simulink model "generic_uservehicle_truck"  (Simulink 10.3)
settings: Solver=ode45  StartTime=0.0  StopTime=inf  RelTol=1e-3  EnableMultiTasking=on
(part 3 of 4)

== system generic_uservehicle_truck/TruckMaker/Vehicle/User Vehicle (CM4SL)/CarAndTrailer/CreateBus Vhcl.Wheel.FL2 ==
  Bus Creator3 : BusCreator  Inputs=14
  Demux3 : Demux  Outputs=14
      settings: DisplayOption=none
  Ground5 : Ground
  Vhcl.Wheel.FL2 : Outport  VectorParamsAs1DForOutWhenUnconnected=off
  wires:
  Demux3/14 -> Bus Creator3/14  "Vhcl Wheel FL2 Trq_WhlBearing"
  Demux3/13 -> Bus Creator3/13  "Vhcl Wheel FL2 Trq_T2W"
  Demux3/12 -> Bus Creator3/12  "Vhcl Wheel FL2 SideSlip"
  Demux3/11 -> Bus Creator3/11  "Vhcl Wheel FL2 LongSlip"
  Demux3/10 -> Bus Creator3/10  "Vhcl Wheel FL2 vBelt"
  Demux3/9 -> Bus Creator3/9  "Vhcl Wheel FL2 Fz"
  Demux3/8 -> Bus Creator3/8  "Vhcl Wheel FL2 Fy"
  Demux3/7 -> Bus Creator3/7  "Vhcl Wheel FL2 Fx"
  Demux3/6 -> Bus Creator3/6  "Vhcl Wheel FL2 r_zxy z"
  Demux3/5 -> Bus Creator3/5  "Vhcl Wheel FL2 r_zxy y"
  Demux3/4 -> Bus Creator3/4  "Vhcl Wheel FL2 r_zxy x"
  Demux3/3 -> Bus Creator3/3  "Vhcl Wheel FL2 t z"
  Demux3/2 -> Bus Creator3/2  "Vhcl Wheel FL2 t y"
  Demux3/1 -> Bus Creator3/1  "Vhcl Wheel FL2 t x"
  Bus Creator3/1 -> Vhcl.Wheel.FL2/1
  Ground5/1 -> Demux3/1

== system generic_uservehicle_truck/TruckMaker/Vehicle/User Vehicle (CM4SL)/CarAndTrailer/CreateBus Vhcl.Wheel.FR ==
  Demux3 : Demux  Outputs=14
      settings: DisplayOption=none
  Ground4 : Ground
  Mux : Mux  Inputs=14
  Vhcl.Wheel.FR : Outport  VectorParamsAs1DForOutWhenUnconnected=off
  wires:
  Demux3/1 -> Mux/1  "Vhcl Wheel FR t x"
  Mux/1 -> Vhcl.Wheel.FR/1
  Ground4/1 -> Demux3/1
  Demux3/2 -> Mux/2  "Vhcl Wheel FR t y"
  Demux3/3 -> Mux/3  "Vhcl Wheel FR t z"
  Demux3/4 -> Mux/4  "Vhcl Wheel FR r_zxy x"
  Demux3/5 -> Mux/5  "Vhcl Wheel FR r_zxy y"
  Demux3/6 -> Mux/6  "Vhcl Wheel FR r_zxy z"
  Demux3/7 -> Mux/7  "Vhcl Wheel FR Fx"
  Demux3/8 -> Mux/8  "Vhcl Wheel FR Fy"
  Demux3/9 -> Mux/9  "Vhcl Wheel FR Fz"
  Demux3/10 -> Mux/10  "Vhcl Wheel FR vBelt"
  Demux3/11 -> Mux/11  "Vhcl Wheel FR LongSlip"
  Demux3/12 -> Mux/12  "Vhcl Wheel FR SideSlip"
  Demux3/13 -> Mux/13  "Vhcl Wheel FR Trq_T2W"
  Demux3/14 -> Mux/14  "Vhcl Wheel FR Trq_WhlBearing"

== system generic_uservehicle_truck/TruckMaker/Vehicle/User Vehicle (CM4SL)/CarAndTrailer/CreateBus Vhcl.Wheel.FR2 ==
  Bus Creator3 : BusCreator  Inputs=14
  Demux3 : Demux  Outputs=14
      settings: DisplayOption=none
  Ground6 : Ground
  Vhcl.Wheel.FR2 : Outport  VectorParamsAs1DForOutWhenUnconnected=off
  wires:
  Demux3/14 -> Bus Creator3/14  "Vhcl Wheel FR2 Trq_WhlBearing"
  Demux3/13 -> Bus Creator3/13  "Vhcl Wheel FR2 Trq_T2W"
  Demux3/12 -> Bus Creator3/12  "Vhcl Wheel FR2 SideSlip"
  Demux3/11 -> Bus Creator3/11  "Vhcl Wheel FR2 LongSlip"
  Demux3/10 -> Bus Creator3/10  "Vhcl Wheel FR2 vBelt"
  Demux3/9 -> Bus Creator3/9  "Vhcl Wheel FR2 Fz"
  Demux3/8 -> Bus Creator3/8  "Vhcl Wheel FR2 Fy"
  Demux3/7 -> Bus Creator3/7  "Vhcl Wheel FR2 Fx"
  Demux3/6 -> Bus Creator3/6  "Vhcl Wheel FR2 r_zxy z"
  Demux3/5 -> Bus Creator3/5  "Vhcl Wheel FR2 r_zxy y"
  Demux3/4 -> Bus Creator3/4  "Vhcl Wheel FR2 r_zxy x"
  Demux3/3 -> Bus Creator3/3  "Vhcl Wheel FR2 t z"
  Demux3/2 -> Bus Creator3/2  "Vhcl Wheel FR2 t y"
  Demux3/1 -> Bus Creator3/1  "Vhcl Wheel FR2 t x"
  Bus Creator3/1 -> Vhcl.Wheel.FR2/1
  Ground6/1 -> Demux3/1

== system generic_uservehicle_truck/TruckMaker/Vehicle/User Vehicle (CM4SL)/CarAndTrailer/CreateBus Vhcl.Wheel.RL ==
  Demux3 : Demux  Outputs=14
      settings: DisplayOption=none
  Ground5 : Ground
  Mux : Mux  Inputs=14
  Vhcl.Wheel.RL : Outport  VectorParamsAs1DForOutWhenUnconnected=off
  wires:
  Demux3/1 -> Mux/1  "Vhcl Wheel RL t x"
  Mux/1 -> Vhcl.Wheel.RL/1
  Ground5/1 -> Demux3/1
  Demux3/2 -> Mux/2  "Vhcl Wheel RL t y"
  Demux3/3 -> Mux/3  "Vhcl Wheel RL t z"
  Demux3/4 -> Mux/4  "Vhcl Wheel RL r_zxy x"
  Demux3/5 -> Mux/5  "Vhcl Wheel RL r_zxy y"
  Demux3/6 -> Mux/6  "Vhcl Wheel RL r_zxy z"
  Demux3/7 -> Mux/7  "Vhcl Wheel RL Fx"
  Demux3/8 -> Mux/8  "Vhcl Wheel RL Fy"
  Demux3/9 -> Mux/9  "Vhcl Wheel RL Fz"
  Demux3/10 -> Mux/10  "Vhcl Wheel RL vBelt"
  Demux3/11 -> Mux/11  "Vhcl Wheel RL LongSlip"
  Demux3/12 -> Mux/12  "Vhcl Wheel RL SideSlip"
  Demux3/13 -> Mux/13  "Vhcl Wheel RL Trq_T2W"
  Demux3/14 -> Mux/14  "Vhcl Wheel RL Trq_WhlBearing"

== system generic_uservehicle_truck/TruckMaker/Vehicle/User Vehicle (CM4SL)/CarAndTrailer/CreateBus Vhcl.Wheel.RL2 ==
  Bus Creator3 : BusCreator  Inputs=14
  Demux3 : Demux  Outputs=14
      settings: DisplayOption=none
  Ground3 : Ground
  Vhcl.Wheel.RL2 : Outport  VectorParamsAs1DForOutWhenUnconnected=off
  wires:
  Bus Creator3/1 -> Vhcl.Wheel.RL2/1
  Demux3/14 -> Bus Creator3/14  "Vhcl Wheel RL2 Trq_WhlBearing"
  Demux3/13 -> Bus Creator3/13  "Vhcl Wheel RL2 Trq_T2W"
  Demux3/12 -> Bus Creator3/12  "Vhcl Wheel RL2 SideSlip"
  Demux3/11 -> Bus Creator3/11  "Vhcl Wheel RL2 LongSlip"
  Demux3/10 -> Bus Creator3/10  "Vhcl Wheel RL2 vBelt"
  Demux3/9 -> Bus Creator3/9  "Vhcl Wheel RL2 Fz"
  Demux3/8 -> Bus Creator3/8  "Vhcl Wheel RL2 Fy"
  Demux3/7 -> Bus Creator3/7  "Vhcl Wheel RL2 Fx"
  Demux3/6 -> Bus Creator3/6  "Vhcl Wheel RL2 r_zxy z"
  Demux3/5 -> Bus Creator3/5  "Vhcl Wheel RL2 r_zxy y"
  Demux3/4 -> Bus Creator3/4  "Vhcl Wheel RL2 r_zxy x"
  Demux3/3 -> Bus Creator3/3  "Vhcl Wheel RL2 t z"
  Demux3/2 -> Bus Creator3/2  "Vhcl Wheel RL2 t y"
  Demux3/1 -> Bus Creator3/1  "Vhcl Wheel RL2 t x"
  Ground3/1 -> Demux3/1

== system generic_uservehicle_truck/TruckMaker/Vehicle/User Vehicle (CM4SL)/CarAndTrailer/CreateBus Vhcl.Wheel.RL3 ==
  Bus Creator3 : BusCreator  Inputs=14
  Demux3 : Demux  Outputs=14
      settings: DisplayOption=none
  Ground3 : Ground
  Vhcl.Wheel.RL3 : Outport  VectorParamsAs1DForOutWhenUnconnected=off
  wires:
  Ground3/1 -> Demux3/1
  Demux3/1 -> Bus Creator3/1  "Vhcl Wheel RL3 t x"
  Demux3/2 -> Bus Creator3/2  "Vhcl Wheel RL3 t y"
  Demux3/3 -> Bus Creator3/3  "Vhcl Wheel RL3 t z"
  Demux3/4 -> Bus Creator3/4  "Vhcl Wheel RL3 r_zxy x"
  Demux3/5 -> Bus Creator3/5  "Vhcl Wheel RL3 r_zxy y"
  Demux3/6 -> Bus Creator3/6  "Vhcl Wheel RL3 r_zxy z"
  Demux3/7 -> Bus Creator3/7  "Vhcl Wheel RL3 Fx"
  Demux3/8 -> Bus Creator3/8  "Vhcl Wheel RL3 Fy"
  Demux3/9 -> Bus Creator3/9  "Vhcl Wheel RL3 Fz"
  Demux3/10 -> Bus Creator3/10  "Vhcl Wheel RL3 vBelt"
  Demux3/11 -> Bus Creator3/11  "Vhcl Wheel RL3 LongSlip"
  Demux3/12 -> Bus Creator3/12  "Vhcl Wheel RL3 SideSlip"
  Demux3/13 -> Bus Creator3/13  "Vhcl Wheel RL3 Trq_T2W"
  Demux3/14 -> Bus Creator3/14  "Vhcl Wheel RL3 Trq_WhlBearing"
  Bus Creator3/1 -> Vhcl.Wheel.RL3/1

== system generic_uservehicle_truck/TruckMaker/Vehicle/User Vehicle (CM4SL)/CarAndTrailer/CreateBus Vhcl.Wheel.RL4 ==
  Bus Creator3 : BusCreator  Inputs=14
  Demux3 : Demux  Outputs=14
      settings: DisplayOption=none
  Ground3 : Ground
  Vhcl.Wheel.RL4 : Outport  VectorParamsAs1DForOutWhenUnconnected=off
  wires:
  Bus Creator3/1 -> Vhcl.Wheel.RL4/1
  Demux3/14 -> Bus Creator3/14  "Vhcl Wheel RL4 Trq_WhlBearing"
  Demux3/13 -> Bus Creator3/13  "Vhcl Wheel RL4 Trq_T2W"
  Demux3/12 -> Bus Creator3/12  "Vhcl Wheel RL4 SideSlip"
  Demux3/11 -> Bus Creator3/11  "Vhcl Wheel RL4 LongSlip"
  Demux3/10 -> Bus Creator3/10  "Vhcl Wheel RL4 vBelt"
  Demux3/9 -> Bus Creator3/9  "Vhcl Wheel RL4 Fz"
  Demux3/8 -> Bus Creator3/8  "Vhcl Wheel RL4 Fy"
  Demux3/7 -> Bus Creator3/7  "Vhcl Wheel RL4 Fx"
  Demux3/6 -> Bus Creator3/6  "Vhcl Wheel RL4 r_zxy z"
  Demux3/5 -> Bus Creator3/5  "Vhcl Wheel RL4 r_zxy y"
  Demux3/4 -> Bus Creator3/4  "Vhcl Wheel RL4 r_zxy x"
  Demux3/3 -> Bus Creator3/3  "Vhcl Wheel RL4 t z"
  Demux3/2 -> Bus Creator3/2  "Vhcl Wheel RL4 t y"
  Demux3/1 -> Bus Creator3/1  "Vhcl Wheel RL4 t x"
  Ground3/1 -> Demux3/1

== system generic_uservehicle_truck/TruckMaker/Vehicle/User Vehicle (CM4SL)/CarAndTrailer/CreateBus Vhcl.Wheel.RR ==
  Demux3 : Demux  Outputs=14
      settings: DisplayOption=none
  Ground6 : Ground
  Mux : Mux  Inputs=14
  Vhcl.Wheel.RR : Outport  VectorParamsAs1DForOutWhenUnconnected=off
  wires:
  Demux3/1 -> Mux/1  "Vhcl Wheel RR t x"
  Mux/1 -> Vhcl.Wheel.RR/1
  Ground6/1 -> Demux3/1
  Demux3/2 -> Mux/2  "Vhcl Wheel RR t y"
  Demux3/3 -> Mux/3  "Vhcl Wheel RR t z"
  Demux3/4 -> Mux/4  "Vhcl Wheel RR r_zxy x"
  Demux3/5 -> Mux/5  "Vhcl Wheel RR r_zxy y"
  Demux3/6 -> Mux/6  "Vhcl Wheel RR r_zxy z"
  Demux3/7 -> Mux/7  "Vhcl Wheel RR Fx"
  Demux3/8 -> Mux/8  "Vhcl Wheel RR Fy"
  Demux3/9 -> Mux/9  "Vhcl Wheel RR Fz"
  Demux3/10 -> Mux/10  "Vhcl Wheel RR vBelt"
  Demux3/11 -> Mux/11  "Vhcl Wheel RR LongSlip"
  Demux3/12 -> Mux/12  "Vhcl Wheel RR SideSlip"
  Demux3/13 -> Mux/13  "Vhcl Wheel RR Trq_T2W"
  Demux3/14 -> Mux/14  "Vhcl Wheel RR Trq_WhlBearing"

== system generic_uservehicle_truck/TruckMaker/Vehicle/User Vehicle (CM4SL)/CarAndTrailer/CreateBus Vhcl.Wheel.RR2 ==
  Bus Creator3 : BusCreator  Inputs=14
  Demux3 : Demux  Outputs=14
      settings: DisplayOption=none
  Ground4 : Ground
  Vhcl.Wheel.RR2 : Outport  VectorParamsAs1DForOutWhenUnconnected=off
  wires:
  Demux3/14 -> Bus Creator3/14  "Vhcl Wheel RR2 Trq_WhlBearing"
  Demux3/13 -> Bus Creator3/13  "Vhcl Wheel RR2 Trq_T2W"
  Demux3/12 -> Bus Creator3/12  "Vhcl Wheel RR2 SideSlip"
  Demux3/11 -> Bus Creator3/11  "Vhcl Wheel RR2 LongSlip"
  Demux3/10 -> Bus Creator3/10  "Vhcl Wheel RR2 vBelt"
  Demux3/9 -> Bus Creator3/9  "Vhcl Wheel RR2 Fz"
  Demux3/8 -> Bus Creator3/8  "Vhcl Wheel RR2 Fy"
  Demux3/7 -> Bus Creator3/7  "Vhcl Wheel RR2 Fx"
  Demux3/6 -> Bus Creator3/6  "Vhcl Wheel RR2 r_zxy z"
  Demux3/5 -> Bus Creator3/5  "Vhcl Wheel RR2 r_zxy y"
  Demux3/4 -> Bus Creator3/4  "Vhcl Wheel RR2 r_zxy x"
  Demux3/3 -> Bus Creator3/3  "Vhcl Wheel RR2 t z"
  Demux3/2 -> Bus Creator3/2  "Vhcl Wheel RR2 t y"
  Demux3/1 -> Bus Creator3/1  "Vhcl Wheel RR2 t x"
  Bus Creator3/1 -> Vhcl.Wheel.RR2/1
  Ground4/1 -> Demux3/1

== system generic_uservehicle_truck/TruckMaker/Vehicle/User Vehicle (CM4SL)/CarAndTrailer/CreateBus Vhcl.Wheel.RR3 ==
  Bus Creator3 : BusCreator  Inputs=14
  Demux3 : Demux  Outputs=14
      settings: DisplayOption=none
  Ground4 : Ground
  Vhcl.Wheel.RR3 : Outport  VectorParamsAs1DForOutWhenUnconnected=off
  wires:
  Ground4/1 -> Demux3/1
  Bus Creator3/1 -> Vhcl.Wheel.RR3/1
  Demux3/1 -> Bus Creator3/1  "Vhcl Wheel RR3 t x"
  Demux3/2 -> Bus Creator3/2  "Vhcl Wheel RR3 t y"
  Demux3/3 -> Bus Creator3/3  "Vhcl Wheel RR3 t z"
  Demux3/4 -> Bus Creator3/4  "Vhcl Wheel RR3 r_zxy x"
  Demux3/5 -> Bus Creator3/5  "Vhcl Wheel RR3 r_zxy y"
  Demux3/6 -> Bus Creator3/6  "Vhcl Wheel RR3 r_zxy z"
  Demux3/7 -> Bus Creator3/7  "Vhcl Wheel RR3 Fx"
  Demux3/8 -> Bus Creator3/8  "Vhcl Wheel RR3 Fy"
  Demux3/9 -> Bus Creator3/9  "Vhcl Wheel RR3 Fz"
  Demux3/10 -> Bus Creator3/10  "Vhcl Wheel RR3 vBelt"
  Demux3/11 -> Bus Creator3/11  "Vhcl Wheel RR3 LongSlip"
  Demux3/12 -> Bus Creator3/12  "Vhcl Wheel RR3 SideSlip"
  Demux3/13 -> Bus Creator3/13  "Vhcl Wheel RR3 Trq_T2W"
  Demux3/14 -> Bus Creator3/14  "Vhcl Wheel RR3 Trq_WhlBearing"

== system generic_uservehicle_truck/TruckMaker/Vehicle/User Vehicle (CM4SL)/CarAndTrailer/CreateBus Vhcl.Wheel.RR4 ==
  Bus Creator3 : BusCreator  Inputs=14
  Demux3 : Demux  Outputs=14
      settings: DisplayOption=none
  Ground4 : Ground
  Vhcl.Wheel.RR4 : Outport  VectorParamsAs1DForOutWhenUnconnected=off
  wires:
  Demux3/14 -> Bus Creator3/14  "Vhcl Wheel RR4 Trq_WhlBearing"
  Demux3/13 -> Bus Creator3/13  "Vhcl Wheel RR4 Trq_T2W"
  Demux3/12 -> Bus Creator3/12  "Vhcl Wheel RR4 SideSlip"
  Demux3/11 -> Bus Creator3/11  "Vhcl Wheel RR4 LongSlip"
  Demux3/10 -> Bus Creator3/10  "Vhcl Wheel RR4 vBelt"
  Demux3/9 -> Bus Creator3/9  "Vhcl Wheel RR4 Fz"
  Demux3/8 -> Bus Creator3/8  "Vhcl Wheel RR4 Fy"
  Demux3/7 -> Bus Creator3/7  "Vhcl Wheel RR4 Fx"
  Demux3/6 -> Bus Creator3/6  "Vhcl Wheel RR4 r_zxy z"
  Demux3/5 -> Bus Creator3/5  "Vhcl Wheel RR4 r_zxy y"
  Demux3/4 -> Bus Creator3/4  "Vhcl Wheel RR4 r_zxy x"
  Demux3/3 -> Bus Creator3/3  "Vhcl Wheel RR4 t z"
  Demux3/2 -> Bus Creator3/2  "Vhcl Wheel RR4 t y"
  Demux3/1 -> Bus Creator3/1  "Vhcl Wheel RR4 t x"
  Bus Creator3/1 -> Vhcl.Wheel.RR4/1
  Ground4/1 -> Demux3/1

== system generic_uservehicle_truck/TruckMaker/Vehicle/User Vehicle (ModelMgr)/Brake/CreateBus Vhcl.Wheel.PT ==
  In : Inport
  BusCreator : BusCreator  Inputs=60
  Demux : Demux  Outputs=60
      settings: DisplayOption=none
  Out : Outport  VectorParamsAs1DForOutWhenUnconnected=off
  wires:
  Demux/60 -> BusCreator/60  "Vhcl Trq_DriveSrc_trg d11"
  Demux/59 -> BusCreator/59  "Vhcl Trq_DriveSrc_trg d10"
  Demux/58 -> BusCreator/58  "Vhcl Trq_DriveSrc_trg d9"
  Demux/57 -> BusCreator/57  "Vhcl Trq_DriveSrc_trg d8"
  Demux/56 -> BusCreator/56  "Vhcl Trq_DriveSrc_trg d7"
  Demux/55 -> BusCreator/55  "Vhcl Trq_DriveSrc_trg d6"
  Demux/54 -> BusCreator/54  "Vhcl Trq_DriveSrc_trg d5"
  Demux/53 -> BusCreator/53  "Vhcl Trq_DriveSrc_trg d4"
  Demux/52 -> BusCreator/52  "Vhcl Trq_DriveSrc_trg d3"
  Demux/51 -> BusCreator/51  "Vhcl Trq_DriveSrc_trg d2"
  Demux/50 -> BusCreator/50  "Vhcl Trq_DriveSrc_trg d1"
  Demux/49 -> BusCreator/49  "Vhcl Trq_DriveSrc_trg d0"
  Demux/48 -> BusCreator/48  "Vhcl Wheel RR4 WhlBearing"
  Demux/47 -> BusCreator/47  "Vhcl Wheel RR4 Trq_T2W"
  Demux/46 -> BusCreator/46  "Vhcl Wheel RR4 Trq_BrakeReg_trg"
  Demux/45 -> BusCreator/45  "Vhcl Wheel RR4 Trq_Brake"
  Demux/44 -> BusCreator/44  "Vhcl Wheel RL4 WhlBearing"
  Demux/43 -> BusCreator/43  "Vhcl Wheel RL4 Trq_T2W"
  Demux/42 -> BusCreator/42  "Vhcl Wheel RL4 Trq_BrakeReg_trg"
  Demux/41 -> BusCreator/41  "Vhcl Wheel RL4 Trq_Brake"
  Demux/40 -> BusCreator/40  "Vhcl Wheel RR3 WhlBearing"
  Demux/39 -> BusCreator/39  "Vhcl Wheel RR3 Trq_T2W"
  Demux/38 -> BusCreator/38  "Vhcl Wheel RR3 Trq_BrakeReg_trg"
  Demux/37 -> BusCreator/37  "Vhcl Wheel RR3 Trq_Brake"
  Demux/36 -> BusCreator/36  "Vhcl Wheel RL3 WhlBearing"
  Demux/35 -> BusCreator/35  "Vhcl Wheel RL3 Trq_T2W"
  Demux/34 -> BusCreator/34  "Vhcl Wheel RL3 Trq_BrakeReg_trg"
  Demux/33 -> BusCreator/33  "Vhcl Wheel RL3 Trq_Brake"
  Demux/32 -> BusCreator/32  "Vhcl Wheel FR2 WhlBearing"
  Demux/31 -> BusCreator/31  "Vhcl Wheel FR2 Trq_T2W"
  Demux/30 -> BusCreator/30  "Vhcl Wheel FR2 Trq_BrakeReg_trg"
  Demux/29 -> BusCreator/29  "Vhcl Wheel FR2 Trq_Brake"
  Demux/28 -> BusCreator/28  "Vhcl Wheel FL2 WhlBearing"
  Demux/27 -> BusCreator/27  "Vhcl Wheel FL2 Trq_T2W"
  Demux/26 -> BusCreator/26  "Vhcl Wheel FL2 Trq_BrakeReg_trg"
  Demux/25 -> BusCreator/25  "Vhcl Wheel FL2 Trq_Brake"
  Demux/24 -> BusCreator/24  "Vhcl Wheel RR2 WhlBearing"
  Demux/23 -> BusCreator/23  "Vhcl Wheel RR2 Trq_T2W"
  Demux/22 -> BusCreator/22  "Vhcl Wheel RR2 Trq_BrakeReg_trg"
  Demux/21 -> BusCreator/21  "Vhcl Wheel RR2 Trq_Brake"
  Demux/20 -> BusCreator/20  "Vhcl Wheel RL2 WhlBearing"
  Demux/19 -> BusCreator/19  "Vhcl Wheel RL2 Trq_T2W"
  Demux/18 -> BusCreator/18  "Vhcl Wheel RL2 Trq_BrakeReg_trg"
  Demux/17 -> BusCreator/17  "Vhcl Wheel RL2 Trq_Brake"
  Demux/16 -> BusCreator/16  "Vhcl Wheel RR WhlBearing"
  Demux/15 -> BusCreator/15  "Vhcl Wheel RR Trq_T2W"
  Demux/14 -> BusCreator/14  "Vhcl Wheel RR Trq_BrakeReg_trg"
  Demux/13 -> BusCreator/13  "Vhcl Wheel RR Trq_Brake"
  Demux/12 -> BusCreator/12  "Vhcl Wheel RL WhlBearing"
  Demux/11 -> BusCreator/11  "Vhcl Wheel RL Trq_T2W"
  Demux/10 -> BusCreator/10  "Vhcl Wheel RL Trq_BrakeReg_trg"
  Demux/9 -> BusCreator/9  "Vhcl Wheel RL Trq_Brake"
  Demux/8 -> BusCreator/8  "Vhcl Wheel FR WhlBearing"
  Demux/7 -> BusCreator/7  "Vhcl Wheel FR Trq_T2W"
  Demux/6 -> BusCreator/6  "Vhcl Wheel FR Trq_BrakeReg_trg"
  Demux/5 -> BusCreator/5  "Vhcl Wheel FR Trq_Brake"
  Demux/4 -> BusCreator/4  "Vhcl Wheel FL WhlBearing"
  Demux/3 -> BusCreator/3  "Vhcl Wheel FL Trq_T2W"
  Demux/2 -> BusCreator/2  "Vhcl Wheel FL Trq_BrakeReg_trg"
  Demux/1 -> BusCreator/1  "Vhcl Wheel FL Trq_Brake"
  BusCreator/1 -> Out/1
  In/1 -> Demux/1

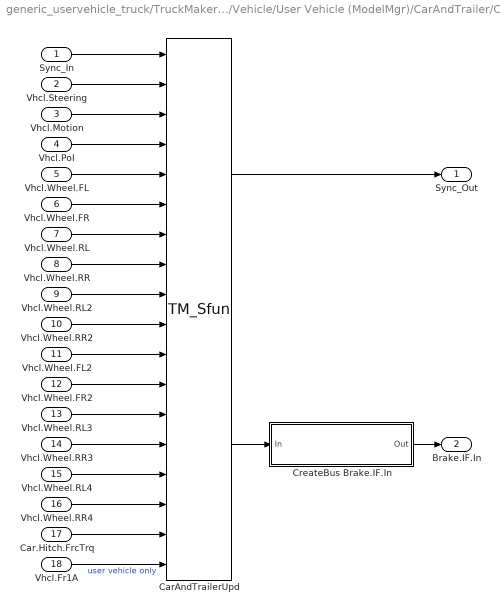
== system generic_uservehicle_truck/TruckMaker/Vehicle/User Vehicle (ModelMgr)/CarAndTrailer/CarAndTrailerUpd ==
  Sync_In : Inport
  Vhcl.Steering : Inport  Port=2
  Vhcl.Motion : Inport  Port=3
  Vhcl.PoI : Inport  Port=4
  Vhcl.Wheel.FL : Inport  Port=5
  Vhcl.Wheel.FR : Inport  Port=6
  Vhcl.Wheel.RL : Inport  Port=7
  Vhcl.Wheel.RR : Inport  Port=8
  Vhcl.Wheel.RL2 : Inport  Port=9
  Vhcl.Wheel.RR2 : Inport  Port=10
  Vhcl.Wheel.FL2 : Inport  Port=11
  Vhcl.Wheel.FR2 : Inport  Port=12
  Vhcl.Wheel.RL3 : Inport  Port=13
  Vhcl.Wheel.RR3 : Inport  Port=14
  Vhcl.Wheel.RL4 : Inport  Port=15
  Vhcl.Wheel.RR4 : Inport  Port=16
  Car.Hitch.FrcTrq : Inport  Port=17
  Vhcl.Fr1A : Inport  Port=18
  CarAndTrailerUpd : S-Function  FunctionName=TM_Sfun  Parameters='CarAndTrUpd'  SFunctionDeploymentMode=off  EnableBusSupport=off
  CreateBus Brake.IF.In : Subsystem
  Sync_Out : Outport  VectorParamsAs1DForOutWhenUnconnected=off
  Brake.IF.In : Outport  Port=2  VectorParamsAs1DForOutWhenUnconnected=off
  wires:
  Vhcl.Wheel.RL3/1 -> CarAndTrailerUpd/13
  Vhcl.Wheel.RR3/1 -> CarAndTrailerUpd/14
  Vhcl.Wheel.RL4/1 -> CarAndTrailerUpd/15
  Vhcl.Wheel.RR4/1 -> CarAndTrailerUpd/16
  Vhcl.Fr1A/1 -> CarAndTrailerUpd/18  "user vehicle only"
  Vhcl.Wheel.RL2/1 -> CarAndTrailerUpd/9
  Vhcl.Wheel.RR2/1 -> CarAndTrailerUpd/10
  Vhcl.Wheel.FL2/1 -> CarAndTrailerUpd/11
  Vhcl.Wheel.FR2/1 -> CarAndTrailerUpd/12
  Car.Hitch.FrcTrq/1 -> CarAndTrailerUpd/17
  Vhcl.Wheel.RR/1 -> CarAndTrailerUpd/8
  Vhcl.Wheel.RL/1 -> CarAndTrailerUpd/7
  Vhcl.Wheel.FR/1 -> CarAndTrailerUpd/6
  Vhcl.Wheel.FL/1 -> CarAndTrailerUpd/5
  Vhcl.Steering/1 -> CarAndTrailerUpd/2
  Vhcl.Motion/1 -> CarAndTrailerUpd/3
  Vhcl.PoI/1 -> CarAndTrailerUpd/4
  CarAndTrailerUpd/2 -> CreateBus Brake.IF.In/1(In)
  CreateBus Brake.IF.In/1(Out) -> Brake.IF.In/1
  CarAndTrailerUpd/1 -> Sync_Out/1
  Sync_In/1 -> CarAndTrailerUpd/1

== system generic_uservehicle_truck/TruckMaker/Vehicle/IPG Vehicle/CarAndTrailer/CarAndTrailerUpd/CreateBus Brake.IF.In ==
  In : Inport
  BusCreator : BusCreator  Inputs=25
  Demux : Demux  Outputs=25
      settings: DisplayOption=none
  Out : Outport  VectorParamsAs1DForOutWhenUnconnected=off
  wires:
  Demux/25 -> BusCreator/25  "Brake IF Trq_Reg RR4"
  Demux/24 -> BusCreator/24  "Brake IF Trq_Reg RL4"
  Demux/23 -> BusCreator/23  "Brake IF Trq_Reg RR3"
  Demux/22 -> BusCreator/22  "Brake IF Trq_Reg RL3"
  Demux/21 -> BusCreator/21  "Brake IF Trq_Reg FR2"
  Demux/20 -> BusCreator/20  "Brake IF Trq_Reg FL2"
  Demux/19 -> BusCreator/19  "Brake IF Trq_Reg RR2"
  Demux/18 -> BusCreator/18  "Brake IF Trq_Reg RL2"
  Demux/17 -> BusCreator/17  "Brake IF Trq_Reg RR"
  Demux/16 -> BusCreator/16  "Brake IF Trq_Reg RL"
  Demux/15 -> BusCreator/15  "Brake IF Trq_Reg FR"
  Demux/14 -> BusCreator/14  "Brake IF Trq_Reg FL"
  Demux/13 -> BusCreator/13  "Brake IF Trq_Reg_max RR4"
  Demux/12 -> BusCreator/12  "Brake IF Trq_Reg_max RL4"
  Demux/11 -> BusCreator/11  "Brake IF Trq_Reg_max RR3"
  Demux/10 -> BusCreator/10  "Brake IF Trq_Reg_max RL3"
  Demux/9 -> BusCreator/9  "Brake IF Trq_Reg_max FR2"
  Demux/8 -> BusCreator/8  "Brake IF Trq_Reg_max FL2"
  Demux/7 -> BusCreator/7  "Brake IF Trq_Reg_max RR2"
  Demux/6 -> BusCreator/6  "Brake IF Trq_Reg_max RL2"
  Demux/5 -> BusCreator/5  "Brake IF Trq_Reg_max RR"
  Demux/4 -> BusCreator/4  "Brake IF Trq_Reg_max RL"
  Demux/3 -> BusCreator/3  "Brake IF Trq_Reg_max FR"
  Demux/2 -> BusCreator/2  "Brake IF Trq_Reg_max FL"
  Demux/1 -> BusCreator/1  "Brake IF T_env"
  BusCreator/1 -> Out/1
  In/1 -> Demux/1

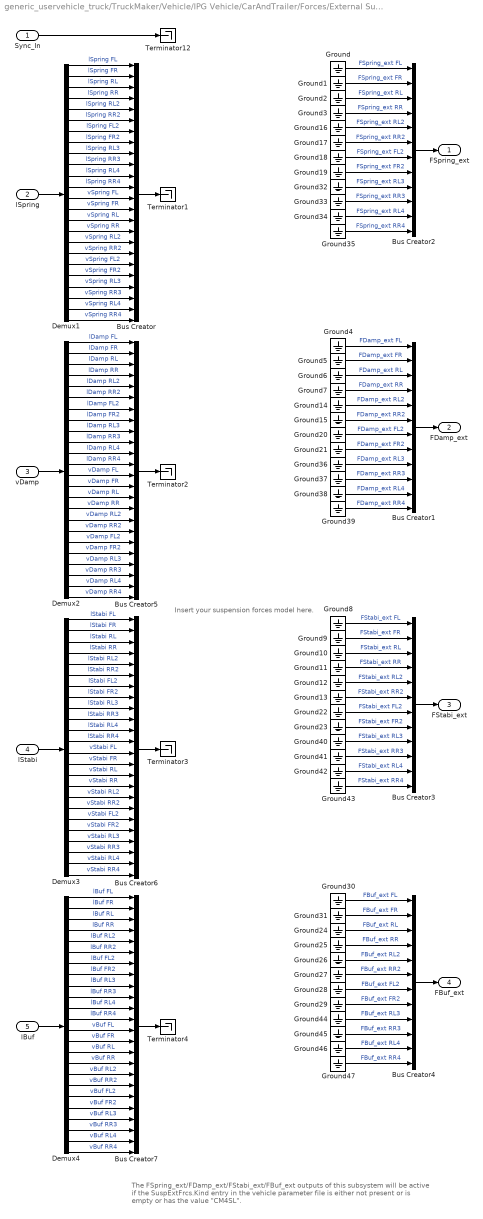
== system generic_uservehicle_truck/TruckMaker/Vehicle/IPG Vehicle/CarAndTrailer/Forces/External Suspension Forces ==
  note: The FSpring_ext/FDamp_ext/FStabi_ext/FBuf_ext outputs of this subsystem will be
      | active if the SuspExtFrcs.Kind entry in the vehicle parameter file
      | is either not present or is empty or has the value "CM4SL".
  note: Insert your suspension forces model here.
  Sync_In : Inport
  lSpring : Inport  Port=2
  vDamp : Inport  Port=3
  lStabi : Inport  Port=4
  lBuf : Inport  Port=5
  Bus Creator{,5..7} (4 alike) : BusCreator  Inputs=24
  Bus Creator{1..4} (4 alike) : BusCreator  Inputs=12
  Demux{1..4} (4 alike) : Demux  Outputs=24
      settings: DisplayOption=none
  Ground{,1..47} (48 alike) : Ground
  Terminator{1..4,12} (5 alike) : Terminator
  FSpring_ext : Outport  VectorParamsAs1DForOutWhenUnconnected=off
  FDamp_ext : Outport  Port=2  VectorParamsAs1DForOutWhenUnconnected=off
  FStabi_ext : Outport  Port=3  VectorParamsAs1DForOutWhenUnconnected=off
  FBuf_ext : Outport  Port=4  VectorParamsAs1DForOutWhenUnconnected=off
  wires:
  Ground46/1 -> Bus Creator4/11  "FBuf_ext RL4"
  Ground47/1 -> Bus Creator4/12  "FBuf_ext RR4"
  Ground45/1 -> Bus Creator4/10  "FBuf_ext RR3"
  Ground44/1 -> Bus Creator4/9  "FBuf_ext RL3"
  Ground42/1 -> Bus Creator3/11  "FStabi_ext RL4"
  Ground43/1 -> Bus Creator3/12  "FStabi_ext RR4"
  Ground41/1 -> Bus Creator3/10  "FStabi_ext RR3"
  Ground40/1 -> Bus Creator3/9  "FStabi_ext RL3"
  Ground38/1 -> Bus Creator1/11  "FDamp_ext RL4"
  Ground39/1 -> Bus Creator1/12  "FDamp_ext RR4"
  Ground37/1 -> Bus Creator1/10  "FDamp_ext RR3"
  Ground36/1 -> Bus Creator1/9  "FDamp_ext RL3"
  Ground35/1 -> Bus Creator2/12  "FSpring_ext RR4"
  Ground34/1 -> Bus Creator2/11  "FSpring_ext RL4"
  Ground33/1 -> Bus Creator2/10  "FSpring_ext RR3"
  Ground32/1 -> Bus Creator2/9  "FSpring_ext RL3"
  Demux4/24 -> Bus Creator7/24  "vBuf RR4"
  Demux4/23 -> Bus Creator7/23  "vBuf RL4"
  Demux4/22 -> Bus Creator7/22  "vBuf RR3"
  Demux4/21 -> Bus Creator7/21  "vBuf RL3"
  Demux4/20 -> Bus Creator7/20  "vBuf FR2"
  Demux4/19 -> Bus Creator7/19  "vBuf FL2"
  Demux4/18 -> Bus Creator7/18  "vBuf RR2"
  Demux4/17 -> Bus Creator7/17  "vBuf RL2"
  Demux3/24 -> Bus Creator6/24  "vStabi RR4"
  Demux3/23 -> Bus Creator6/23  "vStabi RL4"
  Demux3/22 -> Bus Creator6/22  "vStabi RR3"
  Demux3/21 -> Bus Creator6/21  "vStabi RL3"
  Demux3/20 -> Bus Creator6/20  "vStabi FR2"
  Demux3/19 -> Bus Creator6/19  "vStabi FL2"
  Demux3/18 -> Bus Creator6/18  "vStabi RR2"
  Demux3/17 -> Bus Creator6/17  "vStabi RL2"
  Demux2/24 -> Bus Creator5/24  "vDamp RR4"
  Demux2/23 -> Bus Creator5/23  "vDamp RL4"
  Demux2/22 -> Bus Creator5/22  "vDamp RR3"
  Demux2/21 -> Bus Creator5/21  "vDamp RL3"
  Demux2/20 -> Bus Creator5/20  "vDamp FR2"
  Demux2/19 -> Bus Creator5/19  "vDamp FL2"
  Demux2/18 -> Bus Creator5/18  "vDamp RR2"
  Demux2/17 -> Bus Creator5/17  "vDamp RL2"
  Demux1/24 -> Bus Creator/24  "vSpring RR4"
  Demux1/23 -> Bus Creator/23  "vSpring RL4"
  Demux1/22 -> Bus Creator/22  "vSpring RR3"
  Demux1/21 -> Bus Creator/21  "vSpring RL3"
  Demux1/20 -> Bus Creator/20  "vSpring FR2"
  Demux1/19 -> Bus Creator/19  "vSpring FL2"
  Demux1/18 -> Bus Creator/18  "vSpring RR2"
  Demux1/17 -> Bus Creator/17  "vSpring RL2"
  Demux3/10 -> Bus Creator6/10  "lStabi RR3"
  Demux4/16 -> Bus Creator7/16  "vBuf RR"
  Demux4/15 -> Bus Creator7/15  "vBuf RL"
  Demux4/14 -> Bus Creator7/14  "vBuf FR"
  Demux4/13 -> Bus Creator7/13  "vBuf FL"
  Demux4/12 -> Bus Creator7/12  "lBuf RR4"
  Demux4/11 -> Bus Creator7/11  "lBuf RL4"
  Demux4/10 -> Bus Creator7/10  "lBuf RR3"
  Demux4/9 -> Bus Creator7/9  "lBuf RL3"
  Demux3/16 -> Bus Creator6/16  "vStabi RR"
  Demux3/15 -> Bus Creator6/15  "vStabi RL"
  Demux3/14 -> Bus Creator6/14  "vStabi FR"
  Demux3/13 -> Bus Creator6/13  "vStabi FL"
  Demux3/12 -> Bus Creator6/12  "lStabi RR4"
  Demux3/11 -> Bus Creator6/11  "lStabi RL4"
  Demux3/9 -> Bus Creator6/9  "lStabi RL3"
  Bus Creator6/1 -> Terminator3/1
  Bus Creator7/1 -> Terminator4/1
  Bus Creator5/1 -> Terminator2/1
  Bus Creator/1 -> Terminator1/1
  Demux2/16 -> Bus Creator5/16  "vDamp RR"
  Demux2/15 -> Bus Creator5/15  "vDamp RL"
  Demux2/14 -> Bus Creator5/14  "vDamp FR"
  Demux2/13 -> Bus Creator5/13  "vDamp FL"
  Demux2/12 -> Bus Creator5/12  "lDamp RR4"
  Demux2/11 -> Bus Creator5/11  "lDamp RL4"
  Demux2/10 -> Bus Creator5/10  "lDamp RR3"
  Demux2/9 -> Bus Creator5/9  "lDamp RL3"
  Demux1/16 -> Bus Creator/16  "vSpring RR"
  Demux1/15 -> Bus Creator/15  "vSpring RL"
  Demux1/14 -> Bus Creator/14  "vSpring FR"
  Demux1/13 -> Bus Creator/13  "vSpring FL"
  Demux1/12 -> Bus Creator/12  "lSpring RR4"
  Demux1/11 -> Bus Creator/11  "lSpring RL4"
  Demux1/10 -> Bus Creator/10  "lSpring RR3"
  Demux1/9 -> Bus Creator/9  "lSpring RL3"
  Demux3/7 -> Bus Creator6/7  "lStabi FL2"
  Demux3/8 -> Bus Creator6/8  "lStabi FR2"
  Ground22/1 -> Bus Creator3/7  "FStabi_ext FL2"
  Ground23/1 -> Bus Creator3/8  "FStabi_ext FR2"
  Demux2/7 -> Bus Creator5/7  "lDamp FL2"
  Demux2/8 -> Bus Creator5/8  "lDamp FR2"
  Ground20/1 -> Bus Creator1/7  "FDamp_ext FL2"
  Ground21/1 -> Bus Creator1/8  "FDamp_ext FR2"
  Ground18/1 -> Bus Creator2/7  "FSpring_ext FL2"
  Ground19/1 -> Bus Creator2/8  "FSpring_ext FR2"
  Demux1/7 -> Bus Creator/7  "lSpring FL2"
  Demux1/8 -> Bus Creator/8  "lSpring FR2"
  Sync_In/1 -> Terminator12/1
  lSpring/1 -> Demux1/1
  vDamp/1 -> Demux2/1
  lStabi/1 -> Demux3/1
  Demux3/1 -> Bus Creator6/1  "lStabi FL"
  Demux3/2 -> Bus Creator6/2  "lStabi FR"
  Demux3/3 -> Bus Creator6/3  "lStabi RL"
  Demux3/4 -> Bus Creator6/4  "lStabi RR"
  Demux1/1 -> Bus Creator/1  "lSpring FL"
  Demux1/2 -> Bus Creator/2  "lSpring FR"
  Demux1/3 -> Bus Creator/3  "lSpring RL"
  Demux1/4 -> Bus Creator/4  "lSpring RR"
  Demux2/1 -> Bus Creator5/1  "lDamp FL"
  Demux2/2 -> Bus Creator5/2  "lDamp FR"
  Demux2/3 -> Bus Creator5/3  "lDamp RL"
  Demux2/4 -> Bus Creator5/4  "lDamp RR"
  Bus Creator2/1 -> FSpring_ext/1
  Ground/1 -> Bus Creator2/1  "FSpring_ext FL"
  Ground1/1 -> Bus Creator2/2  "FSpring_ext FR"
  Ground2/1 -> Bus Creator2/3  "FSpring_ext RL"
  Ground3/1 -> Bus Creator2/4  "FSpring_ext RR"
  Ground4/1 -> Bus Creator1/1  "FDamp_ext FL"
  Ground5/1 -> Bus Creator1/2  "FDamp_ext FR"
  Ground6/1 -> Bus Creator1/3  "FDamp_ext RL"
  Ground7/1 -> Bus Creator1/4  "FDamp_ext RR"
  Bus Creator1/1 -> FDamp_ext/1
  Ground8/1 -> Bus Creator3/1  "FStabi_ext FL"
  Ground9/1 -> Bus Creator3/2  "FStabi_ext FR"
  Ground10/1 -> Bus Creator3/3  "FStabi_ext RL"
  Ground11/1 -> Bus Creator3/4  "FStabi_ext RR"
  Bus Creator3/1 -> FStabi_ext/1
  Demux3/5 -> Bus Creator6/5  "lStabi RL2"
  Demux3/6 -> Bus Creator6/6  "lStabi RR2"
  Ground12/1 -> Bus Creator3/5  "FStabi_ext RL2"
  Ground13/1 -> Bus Creator3/6  "FStabi_ext RR2"
  Demux2/5 -> Bus Creator5/5  "lDamp RL2"
  Demux2/6 -> Bus Creator5/6  "lDamp RR2"
  Ground14/1 -> Bus Creator1/5  "FDamp_ext RL2"
  Ground15/1 -> Bus Creator1/6  "FDamp_ext RR2"
  Demux1/5 -> Bus Creator/5  "lSpring RL2"
  Demux1/6 -> Bus Creator/6  "lSpring RR2"
  Ground16/1 -> Bus Creator2/5  "FSpring_ext RL2"
  Ground17/1 -> Bus Creator2/6  "FSpring_ext RR2"
  Demux4/7 -> Bus Creator7/7  "lBuf FL2"
  Demux4/8 -> Bus Creator7/8  "lBuf FR2"
  Ground28/1 -> Bus Creator4/7  "FBuf_ext FL2"
  Ground29/1 -> Bus Creator4/8  "FBuf_ext FR2"
  lBuf/1 -> Demux4/1
  Demux4/1 -> Bus Creator7/1  "lBuf FL"
  Demux4/2 -> Bus Creator7/2  "lBuf FR"
  Demux4/3 -> Bus Creator7/3  "lBuf RL"
  Demux4/4 -> Bus Creator7/4  "lBuf RR"
  Ground30/1 -> Bus Creator4/1  "FBuf_ext FL"
  Ground31/1 -> Bus Creator4/2  "FBuf_ext FR"
  Ground24/1 -> Bus Creator4/3  "FBuf_ext RL"
  Ground25/1 -> Bus Creator4/4  "FBuf_ext RR"
  Bus Creator4/1 -> FBuf_ext/1
  Demux4/5 -> Bus Creator7/5  "lBuf RL2"
  Demux4/6 -> Bus Creator7/6  "lBuf RR2"
  Ground26/1 -> Bus Creator4/5  "FBuf_ext RL2"
  Ground27/1 -> Bus Creator4/6  "FBuf_ext RR2"

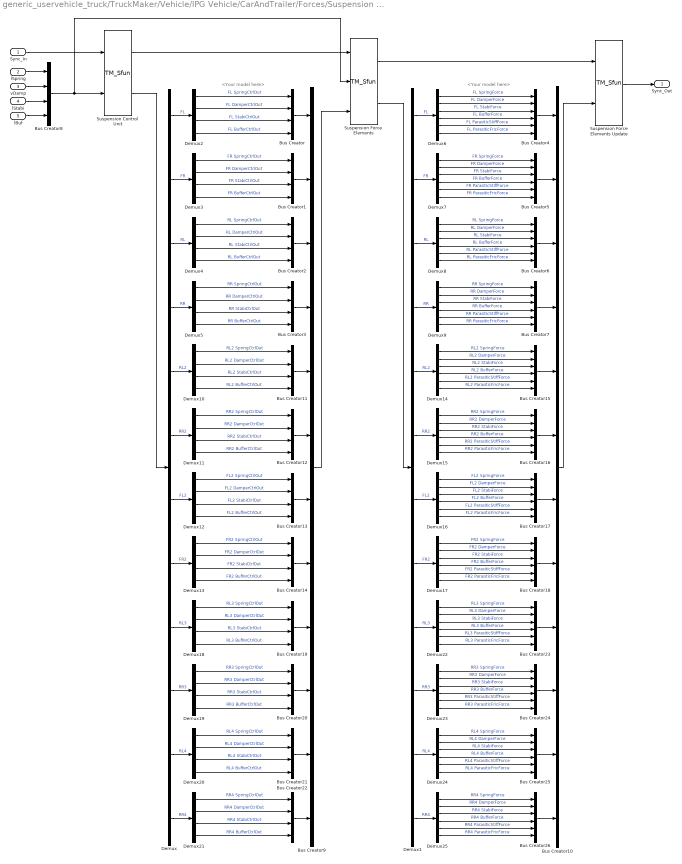
== system generic_uservehicle_truck/TruckMaker/Vehicle/IPG Vehicle/CarAndTrailer/Forces/Suspension Forces ==
  note: <Your model here>
  note: <Your model here>
  Sync_In : Inport
  lSpring : Inport  Port=2
  vDamp : Inport  Port=3
  lStabi : Inport  Port=4
  lBuf : Inport  Port=5
  Bus Creator{,1..3,8,11..14,19..22} (13 alike) : BusCreator  Inputs=4
  Bus Creator10 : BusCreator  Inputs=12
  Bus Creator{4..7,15..18,23..26} (12 alike) : BusCreator  Inputs=6
  Bus Creator9 : BusCreator  Inputs=12
  Demux : Demux  Outputs=12
  Demux1 : Demux  Outputs=12
  Demux{2..5,10..13,18..21} (12 alike) : Demux
  Demux{6..9,14..17,22..25} (12 alike) : Demux  Outputs=6
  Suspension Control Unit : S-Function  FunctionName=TM_Sfun  Parameters='ForcesSuspControl'  SFunctionDeploymentMode=off  EnableBusSupport=off
  Suspension Force Elements : S-Function  FunctionName=TM_Sfun  Parameters='ForcesSusp'  SFunctionDeploymentMode=off  EnableBusSupport=off
  Suspension Force Elements Update : S-Function  FunctionName=TM_Sfun  Parameters='ForcesSuspUpd'  SFunctionDeploymentMode=off  EnableBusSupport=off
  Sync_Out : Outport  VectorParamsAs1DForOutWhenUnconnected=off
  wires:
  Bus Creator26/1 -> Bus Creator10/12
  Bus Creator25/1 -> Bus Creator10/11
  Bus Creator24/1 -> Bus Creator10/10
  Bus Creator23/1 -> Bus Creator10/9
  Demux1/12 -> Demux25/1  "RR4"
  Demux1/11 -> Demux24/1  "RL4"
  Demux1/10 -> Demux23/1  "RR3"
  Demux1/9 -> Demux22/1  "RL3"
  Demux24/6 -> Bus Creator25/6  "RL4 ParasiticFricForce"
  Demux24/5 -> Bus Creator25/5  "RL4 ParasiticStiffForce"
  Demux24/4 -> Bus Creator25/4  "RL4 BufferForce"
  Demux24/3 -> Bus Creator25/3  "RL4 StabiForce"
  Demux24/2 -> Bus Creator25/2  "RL4 DamperForce"
  Demux25/6 -> Bus Creator26/6  "RR4 ParasiticFricForce"
  Demux25/5 -> Bus Creator26/5  "RR4 ParasiticStiffForce"
  Demux25/4 -> Bus Creator26/4  "RR4 BufferForce"
  Demux25/3 -> Bus Creator26/3  "RR4 StabiForce"
  Demux25/2 -> Bus Creator26/2  "RR4 DamperForce"
  Demux25/1 -> Bus Creator26/1  "RR4 SpringForce"
  Demux24/1 -> Bus Creator25/1  "RL4 SpringForce"
  Demux22/1 -> Bus Creator23/1  "RL3 SpringForce"
  Demux23/1 -> Bus Creator24/1  "RR3 SpringForce"
  Demux23/2 -> Bus Creator24/2  "RR3 DamperForce"
  Demux23/3 -> Bus Creator24/3  "RR3 StabiForce"
  Demux23/4 -> Bus Creator24/4  "RR3 BufferForce"
  Demux23/5 -> Bus Creator24/5  "RR3 ParasiticStiffForce"
  Demux23/6 -> Bus Creator24/6  "RR3 ParasiticFricForce"
  Demux22/2 -> Bus Creator23/2  "RL3 DamperForce"
  Demux22/3 -> Bus Creator23/3  "RL3 StabiForce"
  Demux22/4 -> Bus Creator23/4  "RL3 BufferForce"
  Demux22/5 -> Bus Creator23/5  "RL3 ParasiticStiffForce"
  Demux22/6 -> Bus Creator23/6  "RL3 ParasiticFricForce"
  Demux/12 -> Demux21/1  "RR4"
  Demux/11 -> Demux20/1  "RL4"
  Bus Creator21/1 -> Bus Creator9/11
  Demux20/4 -> Bus Creator21/4  "RL4 BufferCtrlOut"
  Demux20/3 -> Bus Creator21/3  "RL4 StabiCtrlOut"
  Demux20/2 -> Bus Creator21/2  "RL4 DamperCtrlOut"
  Demux21/4 -> Bus Creator22/4  "RR4 BufferCtrlOut"
  Demux21/3 -> Bus Creator22/3  "RR4 StabiCtrlOut"
  Demux21/2 -> Bus Creator22/2  "RR4 DamperCtrlOut"
  Demux21/1 -> Bus Creator22/1  "RR4 SpringCtrlOut"
  Demux20/1 -> Bus Creator21/1  "RL4 SpringCtrlOut"
  Bus Creator22/1 -> Bus Creator9/12
  Demux/9 -> Demux18/1  "RL3"
  Bus Creator20/1 -> Bus Creator9/10
  Demux/10 -> Demux19/1  "RR3"
  Demux18/1 -> Bus Creator19/1  "RL3 SpringCtrlOut"
  Demux19/1 -> Bus Creator20/1  "RR3 SpringCtrlOut"
  Demux19/2 -> Bus Creator20/2  "RR3 DamperCtrlOut"
  Demux19/3 -> Bus Creator20/3  "RR3 StabiCtrlOut"
  Demux19/4 -> Bus Creator20/4  "RR3 BufferCtrlOut"
  Demux18/2 -> Bus Creator19/2  "RL3 DamperCtrlOut"
  Demux18/3 -> Bus Creator19/3  "RL3 StabiCtrlOut"
  Demux18/4 -> Bus Creator19/4  "RL3 BufferCtrlOut"
  Bus Creator19/1 -> Bus Creator9/9
  Demux1/8 -> Demux17/1  "FR2"
  Demux1/7 -> Demux16/1  "FL2"
  Demux1/6 -> Demux15/1  "RR2"
  Demux1/5 -> Demux14/1  "RL2"
  Demux14/6 -> Bus Creator15/6  "RL2 ParasiticFricForce"
  Demux14/5 -> Bus Creator15/5  "RL2 ParasiticStiffForce"
  Demux14/4 -> Bus Creator15/4  "RL2 BufferForce"
  Demux14/3 -> Bus Creator15/3  "RL2 StabiForce"
  Demux14/2 -> Bus Creator15/2  "RL2 DamperForce"
  Demux15/6 -> Bus Creator16/6  "RR2 ParasiticFricForce"
  Demux15/5 -> Bus Creator16/5  "RR2 ParasiticStiffForce"
  Demux15/4 -> Bus Creator16/4  "RR2 BufferForce"
  Demux15/3 -> Bus Creator16/3  "RR2 StabiForce"
  Demux15/2 -> Bus Creator16/2  "RR2 DamperForce"
  Demux15/1 -> Bus Creator16/1  "RR2 SpringForce"
  Demux16/3 -> Bus Creator17/3  "FL2 StabiForce"
  Demux16/6 -> Bus Creator17/6  "FL2 ParasiticFricForce"
  Demux16/5 -> Bus Creator17/5  "FL2 ParasiticStiffForce"
  Demux16/4 -> Bus Creator17/4  "FL2 BufferForce"
  Demux16/2 -> Bus Creator17/2  "FL2 DamperForce"
  Demux16/1 -> Bus Creator17/1  "FL2 SpringForce"
  Demux17/6 -> Bus Creator18/6  "FR2 ParasiticFricForce"
  Demux17/5 -> Bus Creator18/5  "FR2 ParasiticStiffForce"
  Demux17/4 -> Bus Creator18/4  "FR2 BufferForce"
  Demux17/3 -> Bus Creator18/3  "FR2 StabiForce"
  Demux17/2 -> Bus Creator18/2  "FR2 DamperForce"
  Demux17/1 -> Bus Creator18/1  "FR2 SpringForce"
  Demux14/1 -> Bus Creator15/1  "RL2 SpringForce"
  Bus Creator18/1 -> Bus Creator10/8
  Bus Creator17/1 -> Bus Creator10/7
  Bus Creator16/1 -> Bus Creator10/6
  Bus Creator15/1 -> Bus Creator10/5
  Bus Creator11/1 -> Bus Creator9/5
  Demux10/4 -> Bus Creator11/4  "RL2 BufferCtrlOut"
  Demux10/3 -> Bus Creator11/3  "RL2 StabiCtrlOut"
  Demux10/2 -> Bus Creator11/2  "RL2 DamperCtrlOut"
  Demux11/4 -> Bus Creator12/4  "RR2 BufferCtrlOut"
  Demux11/3 -> Bus Creator12/3  "RR2 StabiCtrlOut"
  Demux11/2 -> Bus Creator12/2  "RR2 DamperCtrlOut"
  Demux11/1 -> Bus Creator12/1  "RR2 SpringCtrlOut"
  Demux12/3 -> Bus Creator13/3  "FL2 StabiCtrlOut"
  Demux12/4 -> Bus Creator13/4  "FL2 BufferCtrlOut"
  Demux12/2 -> Bus Creator13/2  "FL2 DamperCtrlOut"
  Demux12/1 -> Bus Creator13/1  "FL2 SpringCtrlOut"
  Demux13/4 -> Bus Creator14/4  "FR2 BufferCtrlOut"
  Demux13/3 -> Bus Creator14/3  "FR2 StabiCtrlOut"
  Demux13/2 -> Bus Creator14/2  "FR2 DamperCtrlOut"
  Demux13/1 -> Bus Creator14/1  "FR2 SpringCtrlOut"
  Demux/8 -> Demux13/1  "FR2"
  Demux10/1 -> Bus Creator11/1  "RL2 SpringCtrlOut"
  Bus Creator14/1 -> Bus Creator9/8
  Demux/7 -> Demux12/1  "FL2"
  Bus Creator13/1 -> Bus Creator9/7
  Demux/6 -> Demux11/1  "RR2"
  Bus Creator12/1 -> Bus Creator9/6
  Demux/5 -> Demux10/1  "RL2"
  Demux1/4 -> Demux9/1  "RR"
  Demux1/3 -> Demux8/1  "RL"
  Demux1/2 -> Demux7/1  "FR"
  Demux1/1 -> Demux6/1  "FL"
  Suspension Force Elements/2 -> Demux1/1
  Bus Creator/1 -> Bus Creator9/1
  Bus Creator9/1 -> Suspension Force Elements/3
  Suspension Control Unit/2 -> Demux/1
  Demux2/4 -> Bus Creator/4  "FL BufferCtrlOut"
  Demux2/3 -> Bus Creator/3  "FL StabiCtrlOut"
  Demux2/2 -> Bus Creator/2  "FL DamperCtrlOut"
  Demux3/4 -> Bus Creator1/4  "FR BufferCtrlOut"
  Demux3/3 -> Bus Creator1/3  "FR StabiCtrlOut"
  Demux3/2 -> Bus Creator1/2  "FR DamperCtrlOut"
  Demux3/1 -> Bus Creator1/1  "FR SpringCtrlOut"
  Demux4/3 -> Bus Creator2/3  "RL StabiCtrlOut"
  Demux4/4 -> Bus Creator2/4  "RL BufferCtrlOut"
  Demux4/2 -> Bus Creator2/2  "RL DamperCtrlOut"
  Demux4/1 -> Bus Creator2/1  "RL SpringCtrlOut"
  Demux5/4 -> Bus Creator3/4  "RR BufferCtrlOut"
  Demux5/3 -> Bus Creator3/3  "RR StabiCtrlOut"
  Demux5/2 -> Bus Creator3/2  "RR DamperCtrlOut"
  Demux5/1 -> Bus Creator3/1  "RR SpringCtrlOut"
  Demux/4 -> Demux5/1  "RR"
  Demux2/1 -> Bus Creator/1  "FL SpringCtrlOut"
  Bus Creator3/1 -> Bus Creator9/4
  Demux/3 -> Demux4/1  "RL"
  Bus Creator2/1 -> Bus Creator9/3
  Demux/2 -> Demux3/1  "FR"
  Bus Creator1/1 -> Bus Creator9/2
  Demux/1 -> Demux2/1  "FL"
  Bus Creator10/1 -> Suspension Force Elements Update/2
  Demux6/6 -> Bus Creator4/6  "FL ParasiticFricForce"
  Demux6/5 -> Bus Creator4/5  "FL ParasiticStiffForce"
  Demux6/4 -> Bus Creator4/4  "FL BufferForce"
  Demux6/3 -> Bus Creator4/3  "FL StabiForce"
  Demux6/2 -> Bus Creator4/2  "FL DamperForce"
  Demux7/6 -> Bus Creator5/6  "FR ParasiticFricForce"
  Demux7/5 -> Bus Creator5/5  "FR ParasiticStiffForce"
  Demux7/4 -> Bus Creator5/4  "FR BufferForce"
  Demux7/3 -> Bus Creator5/3  "FR StabiForce"
  Demux7/2 -> Bus Creator5/2  "FR DamperForce"
  Demux7/1 -> Bus Creator5/1  "FR SpringForce"
  Demux8/3 -> Bus Creator6/3  "RL StabiForce"
  Demux8/6 -> Bus Creator6/6  "RL ParasiticFricForce"
  Demux8/5 -> Bus Creator6/5  "RL ParasiticStiffForce"
  Demux8/4 -> Bus Creator6/4  "RL BufferForce"
  Demux8/2 -> Bus Creator6/2  "RL DamperForce"
  Demux8/1 -> Bus Creator6/1  "RL SpringForce"
  Demux9/6 -> Bus Creator7/6  "RR ParasiticFricForce"
  Demux9/5 -> Bus Creator7/5  "RR ParasiticStiffForce"
  Demux9/4 -> Bus Creator7/4  "RR BufferForce"
  Demux9/3 -> Bus Creator7/3  "RR StabiForce"
  Demux9/2 -> Bus Creator7/2  "RR DamperForce"
  Demux9/1 -> Bus Creator7/1  "RR SpringForce"
  Demux6/1 -> Bus Creator4/1  "FL SpringForce"
  Bus Creator7/1 -> Bus Creator10/4
  Bus Creator6/1 -> Bus Creator10/3
  Bus Creator5/1 -> Bus Creator10/2
  Bus Creator4/1 -> Bus Creator10/1
  Suspension Force Elements Update/1 -> Sync_Out/1
  Suspension Force Elements/1 -> Suspension Force Elements Update/1
  Suspension Control Unit/1 -> Suspension Force Elements/1
  Sync_In/1 -> Suspension Control Unit/1
  Bus Creator8/1 -> Suspension Force Elements/2, Suspension Control Unit/2
  lSpring/1 -> Bus Creator8/1
  lBuf/1 -> Bus Creator8/4
  lStabi/1 -> Bus Creator8/3
  vDamp/1 -> Bus Creator8/2

== system generic_uservehicle_truck/TruckMaker/Vehicle/IPG Vehicle/CarAndTrailer/Forces/Vehicle Forces ==
  Sync_In : Inport
  Bus Creator1 : BusCreator  Inputs=12
  Bus Creator8 : BusCreator  Inputs=16
  BusCreator1 : BusCreator  Inputs=4
  BusCreator2 : BusCreator  Inputs=9
  Demux : Demux  Outputs=16
      settings: DisplayOption=none
  Demux1 : Demux  Outputs=12
      settings: DisplayOption=none
  Demux2 : Demux  Outputs=13
      settings: DisplayOption=none
  Forces : S-Function  FunctionName=TM_Sfun  Parameters='Forces'  SFunctionDeploymentMode=off  EnableBusSupport=off
  Terminator : Terminator
  Sync_Out : Outport  VectorParamsAs1DForOutWhenUnconnected=off
  Car.Virtual : Outport  Port=2  VectorParamsAs1DForOutWhenUnconnected=off
  Car.Aero : Outport  Port=3  VectorParamsAs1DForOutWhenUnconnected=off
  Car.Load : Outport  Port=4  VectorParamsAs1DForOutWhenUnconnected=off
  wires:
  BusCreator1/1 -> Terminator/1  "Aero IF (in)"
  Demux2/13 -> BusCreator2/9  "car Aero Trq_1 z"
  Demux2/12 -> BusCreator2/8  "car Aero Trq_1 y"
  Demux2/11 -> BusCreator2/7  "car Aero Trq_1 x"
  Demux2/10 -> BusCreator2/6  "car Aero Frc_1 z"
  Demux2/9 -> BusCreator2/5  "car Aero Frc_1 y"
  Demux2/8 -> BusCreator2/4  "car Aero Frc_1 x"
  Demux2/7 -> BusCreator2/3  "car Aero PoA_1 z"
  Demux2/6 -> BusCreator2/2  "car Aero PoA_1 y"
  Demux2/5 -> BusCreator2/1  "car Aero PoA_1 x"
  Demux2/4 -> BusCreator1/4  "car Aero tau_1"
  Demux2/3 -> BusCreator1/3  "car Aero ApproachVel_1 z"
  Demux2/2 -> BusCreator1/2  "car Aero ApproachVel_1 y"
  Demux2/1 -> BusCreator1/1  "car Aero ApproachVel_1 x"
  BusCreator2/1 -> Car.Aero/1
  Demux/16 -> Bus Creator8/16  "Car Load_3 tz"
  Demux/15 -> Bus Creator8/15  "Car Load_3 ty"
  Demux/14 -> Bus Creator8/14  "Car Load_3 tx"
  Demux/13 -> Bus Creator8/13  "Car Load_3 mass"
  Demux1/12 -> Bus Creator1/12  "Car Virtual Trq_0 z"
  Demux1/11 -> Bus Creator1/11  "Car Virtual Trq_0 y"
  Demux1/10 -> Bus Creator1/10  "Car Virtual Trq_0 x"
  Demux1/9 -> Bus Creator1/9  "Car Virtual Trq_1 z"
  Demux1/8 -> Bus Creator1/8  "Car Virtual Trq_1 y"
  Demux1/7 -> Bus Creator1/7  "Car Virtual Trq_1 x"
  Demux1/6 -> Bus Creator1/6  "Car Virtual Frc_0 z"
  Demux1/5 -> Bus Creator1/5  "Car Virtual Frc_0 y"
  Demux1/4 -> Bus Creator1/4  "Car Virtual Frc_0 x"
  Sync_In/1 -> Forces/1
  Forces/1 -> Sync_Out/1
  Demux1/1 -> Bus Creator1/1  "Car Virtual Frc_1 x"
  Demux1/2 -> Bus Creator1/2  "Car Virtual Frc_1 y"
  Demux1/3 -> Bus Creator1/3  "Car Virtual Frc_1 z"
  Forces/3 -> Demux2/1
  Forces/2 -> Demux1/1
  Bus Creator1/1 -> Car.Virtual/1
  Bus Creator8/1 -> Car.Load/1
  Demux/1 -> Bus Creator8/1  "Car Load_0 mass"
  Demux/2 -> Bus Creator8/2  "Car Load_0 tx"
  Demux/3 -> Bus Creator8/3  "Car Load_0 ty"
  Demux/4 -> Bus Creator8/4  "Car Load_0 tz"
  Demux/5 -> Bus Creator8/5  "Car Load_1 mass"
  Demux/6 -> Bus Creator8/6  "Car Load_1 tx"
  Demux/7 -> Bus Creator8/7  "Car Load_1 ty"
  Demux/8 -> Bus Creator8/8  "Car Load_1 tz"
  Demux/9 -> Bus Creator8/9  "Car Load_2 mass"
  Demux/10 -> Bus Creator8/10  "Car Load_2 tx"
  Demux/11 -> Bus Creator8/11  "Car Load_2 ty"
  Demux/12 -> Bus Creator8/12  "Car Load_2 tz"
  Forces/4 -> Demux/1

== system generic_uservehicle_truck/TruckMaker/Vehicle/IPG Vehicle/CarAndTrailer/Trailer/CreateBus Car.Hitch.FrcTrq ==
  In1 : Inport
  Bus Creator7 : BusCreator  Inputs=6
  Demux7 : Demux  Outputs=6
      settings: DisplayOption=none
  Out1 : Outport  VectorParamsAs1DForOutWhenUnconnected=off
  wires:
  In1/1 -> Demux7/1
  Bus Creator7/1 -> Out1/1
  Demux7/6 -> Bus Creator7/6  "Car Hitch Trq2Car z"
  Demux7/5 -> Bus Creator7/5  "Car Hitch Trq2Car y"
  Demux7/4 -> Bus Creator7/4  "Car Hitch Trq2Car x"
  Demux7/3 -> Bus Creator7/3  "Car Hitch Frc2Car z"
  Demux7/2 -> Bus Creator7/2  "Car Hitch Frc2Car y"
  Demux7/1 -> Bus Creator7/1  "Car Hitch Frc2Car x"

== system generic_uservehicle_truck/TruckMaker/Vehicle/IPG Vehicle/CarAndTrailer/Trailer/CreateBus Vhcl.Motion ==
  In1 : Inport
  BusCreator : BusCreator  Inputs=15
  Demux : Demux  Outputs=15
      settings: DisplayOption=none
  Out1 : Outport  VectorParamsAs1DForOutWhenUnconnected=off
  wires:
  Demux/15 -> BusCreator/15  "Vhcl YawAcc"
  Demux/14 -> BusCreator/14  "Vhcl YawVel"
  Demux/13 -> BusCreator/13  "Vhcl Yaw"
  Demux/12 -> BusCreator/12  "Vhcl PitchAcc"
  Demux/11 -> BusCreator/11  "Vhcl PitchVel"
  Demux/10 -> BusCreator/10  "Vhcl Pitch"
  Demux/9 -> BusCreator/9  "Vhcl RollAcc"
  Demux/8 -> BusCreator/8  "Vhcl RollVel"
  Demux/7 -> BusCreator/7  "Vhcl Roll"
  Demux/6 -> BusCreator/6  "Vhcl Hitch_Pos z"
  Demux/5 -> BusCreator/5  "Vhcl Hitch_Pos y"
  Demux/4 -> BusCreator/4  "Vhcl Hitch_Pos x"
  Demux/3 -> BusCreator/3  "Vhcl sRoad"
  Demux/2 -> BusCreator/2  "Vhcl Distance"
  Demux/1 -> BusCreator/1  "Vhcl v"
  In1/1 -> Demux/1
  BusCreator/1 -> Out1/1

== system generic_uservehicle_truck/TruckMaker/Vehicle/IPG Vehicle/CarAndTrailer/Trailer/CreateBus Vhcl.PoI ==
  In1 : Inport
  Bus Creator3 : BusCreator  Inputs=18
  Demux3 : Demux  Outputs=18
      settings: DisplayOption=none
  Out1 : Outport  VectorParamsAs1DForOutWhenUnconnected=off
  wires:
  Demux3/18 -> Bus Creator3/18  "Vhcl PoI_GCS Elev"
  Demux3/17 -> Bus Creator3/17  "Vhcl PoI_GCS Lat"
  Demux3/16 -> Bus Creator3/16  "Vhcl PoI_GCS Long"
  Demux3/15 -> Bus Creator3/15  "Vhcl PoI_Acc_1 z"
  Demux3/14 -> Bus Creator3/14  "Vhcl PoI_Acc_1 y"
  Demux3/13 -> Bus Creator3/13  "Vhcl PoI_Acc_1 x"
  Demux3/12 -> Bus Creator3/12  "Vhcl PoI_Vel_1 z"
  Demux3/11 -> Bus Creator3/11  "Vhcl PoI_Vel_1 y"
  Demux3/10 -> Bus Creator3/10  "Vhcl PoI_Vel_1 x"
  Demux3/9 -> Bus Creator3/9  "Vhcl PoI_Acc z"
  Demux3/8 -> Bus Creator3/8  "Vhcl PoI_Acc y"
  Demux3/7 -> Bus Creator3/7  "Vhcl PoI_Acc x"
  Demux3/6 -> Bus Creator3/6  "Vhcl PoI_Vel z"
  Demux3/5 -> Bus Creator3/5  "Vhcl PoI_Vel y"
  Demux3/4 -> Bus Creator3/4  "Vhcl PoI_Vel x"
  Demux3/3 -> Bus Creator3/3  "Vhcl PoI_Pos z"
  Demux3/2 -> Bus Creator3/2  "Vhcl PoI_Pos y"
  In1/1 -> Demux3/1
  Bus Creator3/1 -> Out1/1
  Demux3/1 -> Bus Creator3/1  "Vhcl PoI_Pos x"

== system generic_uservehicle_truck/TruckMaker/Vehicle/IPG Vehicle/CarAndTrailer/Trailer/CreateBus Vhcl.Steering ==
  In1 : Inport
  Bus Creator3 : BusCreator  Inputs=4
  Demux : Demux
      settings: DisplayOption=none
  Out1 : Outport  VectorParamsAs1DForOutWhenUnconnected=off
  wires:
  Bus Creator3/1 -> Out1/1
  Demux/1 -> Bus Creator3/1  "Vhcl Steering Ang"
  Demux/3 -> Bus Creator3/3  "Vhcl Steering AngAcc"
  Demux/2 -> Bus Creator3/2  "Vhcl Steering AngVel"
  Demux/4 -> Bus Creator3/4  "Vhcl Steering Trq"
  In1/1 -> Demux/1

== system generic_uservehicle_truck/TruckMaker/Vehicle/IPG Vehicle/CarAndTrailer/Trailer/CreateBus Vhcl.Wheel.FL ==
  In1 : Inport
  Bus Creator3 : BusCreator  Inputs=14
  Demux3 : Demux  Outputs=14
      settings: DisplayOption=none
  Out1 : Outport  VectorParamsAs1DForOutWhenUnconnected=off
  wires:
  Demux3/14 -> Bus Creator3/14  "Vhcl Wheel FL Trq_WhlBearing"
  Demux3/13 -> Bus Creator3/13  "Vhcl Wheel FL Trq_T2W"
  Demux3/12 -> Bus Creator3/12  "Vhcl Wheel FL SideSlip"
  Demux3/11 -> Bus Creator3/11  "Vhcl Wheel FL LongSlip"
  Demux3/10 -> Bus Creator3/10  "Vhcl Wheel FL vBelt"
  Demux3/9 -> Bus Creator3/9  "Vhcl Wheel FL Fz"
  Demux3/8 -> Bus Creator3/8  "Vhcl Wheel FL Fy"
  Demux3/7 -> Bus Creator3/7  "Vhcl Wheel FL Fx"
  Demux3/6 -> Bus Creator3/6  "Vhcl Wheel FL r_zxy z"
  Demux3/5 -> Bus Creator3/5  "Vhcl Wheel FL r_zxy y"
  Demux3/4 -> Bus Creator3/4  "Vhcl Wheel FL r_zxy x"
  Demux3/3 -> Bus Creator3/3  "Vhcl Wheel FL t z"
  Demux3/2 -> Bus Creator3/2  "Vhcl Wheel FL t y"
  In1/1 -> Demux3/1
  Bus Creator3/1 -> Out1/1
  Demux3/1 -> Bus Creator3/1  "Vhcl Wheel FL t x"

== system generic_uservehicle_truck/TruckMaker/Vehicle/IPG Vehicle/CarAndTrailer/Trailer/CreateBus Vhcl.Wheel.FL2 ==
  In1 : Inport
  Bus Creator3 : BusCreator  Inputs=14
  Demux3 : Demux  Outputs=14
      settings: DisplayOption=none
  Out1 : Outport  VectorParamsAs1DForOutWhenUnconnected=off
  wires:
  Demux3/14 -> Bus Creator3/14  "Vhcl Wheel FL2 Trq_WhlBearing"
  Demux3/13 -> Bus Creator3/13  "Vhcl Wheel FL2 Trq_T2W"
  Demux3/12 -> Bus Creator3/12  "Vhcl Wheel FL2 SideSlip"
  Demux3/11 -> Bus Creator3/11  "Vhcl Wheel FL2 LongSlip"
  Demux3/10 -> Bus Creator3/10  "Vhcl Wheel FL2 vBelt"
  Demux3/9 -> Bus Creator3/9  "Vhcl Wheel FL2 Fz"
  Demux3/8 -> Bus Creator3/8  "Vhcl Wheel FL2 Fy"
  Demux3/7 -> Bus Creator3/7  "Vhcl Wheel FL2 Fx"
  Demux3/6 -> Bus Creator3/6  "Vhcl Wheel FL2 r_zxy z"
  Demux3/5 -> Bus Creator3/5  "Vhcl Wheel FL2 r_zxy y"
  Demux3/4 -> Bus Creator3/4  "Vhcl Wheel FL2 r_zxy x"
  Demux3/3 -> Bus Creator3/3  "Vhcl Wheel FL2 t z"
  Demux3/2 -> Bus Creator3/2  "Vhcl Wheel FL2 t y"
  In1/1 -> Demux3/1
  Bus Creator3/1 -> Out1/1
  Demux3/1 -> Bus Creator3/1  "Vhcl Wheel FL2 t x"

== system generic_uservehicle_truck/TruckMaker/Vehicle/IPG Vehicle/CarAndTrailer/Trailer/CreateBus Vhcl.Wheel.FR ==
  In1 : Inport
  Bus Creator3 : BusCreator  Inputs=14
  Demux3 : Demux  Outputs=14
      settings: DisplayOption=none
  Out1 : Outport  VectorParamsAs1DForOutWhenUnconnected=off
  wires:
  Demux3/14 -> Bus Creator3/14  "Vhcl Wheel FR Trq_WhlBearing"
  Demux3/13 -> Bus Creator3/13  "Vhcl Wheel FR Trq_T2W"
  Demux3/12 -> Bus Creator3/12  "Vhcl Wheel FR SideSlip"
  Demux3/11 -> Bus Creator3/11  "Vhcl Wheel FR LongSlip"
  Demux3/10 -> Bus Creator3/10  "Vhcl Wheel FR vBelt"
  Demux3/9 -> Bus Creator3/9  "Vhcl Wheel FR Fz"
  Demux3/8 -> Bus Creator3/8  "Vhcl Wheel FR Fy"
  Demux3/7 -> Bus Creator3/7  "Vhcl Wheel FR Fx"
  Demux3/6 -> Bus Creator3/6  "Vhcl Wheel FR r_zxy z"
  Demux3/5 -> Bus Creator3/5  "Vhcl Wheel FR r_zxy y"
  Demux3/4 -> Bus Creator3/4  "Vhcl Wheel FR r_zxy x"
  Demux3/3 -> Bus Creator3/3  "Vhcl Wheel FR t z"
  Demux3/2 -> Bus Creator3/2  "Vhcl Wheel FR t y"
  In1/1 -> Demux3/1
  Bus Creator3/1 -> Out1/1
  Demux3/1 -> Bus Creator3/1  "Vhcl Wheel FR t x"

== system generic_uservehicle_truck/TruckMaker/Vehicle/IPG Vehicle/CarAndTrailer/Trailer/CreateBus Vhcl.Wheel.FR2 ==
  In1 : Inport
  Bus Creator3 : BusCreator  Inputs=14
  Demux3 : Demux  Outputs=14
      settings: DisplayOption=none
  Out1 : Outport  VectorParamsAs1DForOutWhenUnconnected=off
  wires:
  Demux3/14 -> Bus Creator3/14  "Vhcl Wheel FR2 Trq_WhlBearing"
  Demux3/13 -> Bus Creator3/13  "Vhcl Wheel FR2 Trq_T2W"
  Demux3/12 -> Bus Creator3/12  "Vhcl Wheel FR2 SideSlip"
  Demux3/11 -> Bus Creator3/11  "Vhcl Wheel FR2 LongSlip"
  Demux3/10 -> Bus Creator3/10  "Vhcl Wheel FR2 vBelt"
  Demux3/9 -> Bus Creator3/9  "Vhcl Wheel FR2 Fz"
  Demux3/8 -> Bus Creator3/8  "Vhcl Wheel FR2 Fy"
  Demux3/7 -> Bus Creator3/7  "Vhcl Wheel FR2 Fx"
  Demux3/6 -> Bus Creator3/6  "Vhcl Wheel FR2 r_zxy z"
  Demux3/5 -> Bus Creator3/5  "Vhcl Wheel FR2 r_zxy y"
  Demux3/4 -> Bus Creator3/4  "Vhcl Wheel FR2 r_zxy x"
  Demux3/3 -> Bus Creator3/3  "Vhcl Wheel FR2 t z"
  Demux3/2 -> Bus Creator3/2  "Vhcl Wheel FR2 t y"
  In1/1 -> Demux3/1
  Bus Creator3/1 -> Out1/1
  Demux3/1 -> Bus Creator3/1  "Vhcl Wheel FR2 t x"

== system generic_uservehicle_truck/TruckMaker/Vehicle/IPG Vehicle/CarAndTrailer/Trailer/CreateBus Vhcl.Wheel.RL ==
  In1 : Inport
  Bus Creator3 : BusCreator  Inputs=14
  Demux3 : Demux  Outputs=14
      settings: DisplayOption=none
  Out1 : Outport  VectorParamsAs1DForOutWhenUnconnected=off
  wires:
  Demux3/14 -> Bus Creator3/14  "Vhcl Wheel RL Trq_WhlBearing"
  Demux3/13 -> Bus Creator3/13  "Vhcl Wheel RL Trq_T2W"
  Demux3/12 -> Bus Creator3/12  "Vhcl Wheel RL SideSlip"
  Demux3/11 -> Bus Creator3/11  "Vhcl Wheel RL LongSlip"
  Demux3/10 -> Bus Creator3/10  "Vhcl Wheel RL vBelt"
  Demux3/9 -> Bus Creator3/9  "Vhcl Wheel RL Fz"
  Demux3/8 -> Bus Creator3/8  "Vhcl Wheel RL Fy"
  Demux3/7 -> Bus Creator3/7  "Vhcl Wheel RL Fx"
  Demux3/6 -> Bus Creator3/6  "Vhcl Wheel RL r_zxy z"
  Demux3/5 -> Bus Creator3/5  "Vhcl Wheel RL r_zxy y"
  Demux3/4 -> Bus Creator3/4  "Vhcl Wheel RL r_zxy x"
  Demux3/3 -> Bus Creator3/3  "Vhcl Wheel RL t z"
  Demux3/2 -> Bus Creator3/2  "Vhcl Wheel RL t y"
  In1/1 -> Demux3/1
  Bus Creator3/1 -> Out1/1
  Demux3/1 -> Bus Creator3/1  "Vhcl Wheel RL t x"
